simulink model "gm_current_fpga_slrt"  (R2020b)
settings: Solver=FixedStepAuto  StartTime=0.0  StopTime=10.0  RelTol=1e-3
undefined symbols (not defined in the file): current_fpga, FPGA, IO334
libraries: speedgoatlib_hdlCoder_IO3xx x5
settings Model: SimulationMode=external  Creator=Student  LastModifiedBy=Student
settings SolverCC: ConcurrentTasks=on  PositivePriorityOrder=on
settings OptimizationCC: BlockReduction=off  ConditionallyExecuteInputs=off  DefaultParameterBehavior=Inlined  OptimizeBlockIOStorage=off
settings DebuggingCC: AlgebraicLoopMsg=error  TasksWithSamePriorityMsg=none
settings HardwareCC: ProdBitPerLong=64  ProdLongLongMode=on  ProdHWDeviceType=Intel->x86-64 (Linux 64)  TargetBitPerPointer=64  TargetBitPerSizeT=64  TargetBitPerPtrDiffT=64  TargetLongLongMode=on  TargetIntDivRoundTo=Zero  TargetEndianess=LittleEndian  TargetWordSize=64  TargetHWDeviceType=Custom Processor->MATLAB Host Computer
settings RTWCC: Description=Simulink Real-Time  SystemTargetFile=slrealtime.tlc  TemplateMakefile=slrealtime_default_tmf  Toolchain=Simulink Real-Time Toolchain  BuildConfiguration=Faster Runs  CodeExecutionProfiling=on  TargetLang=C++

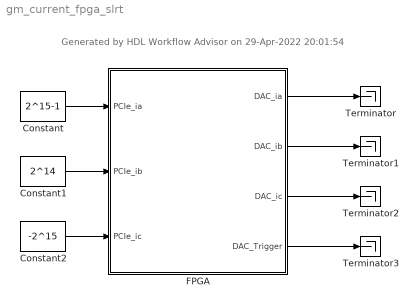
== system gm_current_fpga_slrt ==
  note: Generated by HDL Workflow Advisor on 29-Apr-2022 20:01:54
  Constant : Constant  Value=2^15-1  OutDataTypeStr=int16  SampleTime=5e-5
  Constant1 : Constant  Value=2^14  OutDataTypeStr=int16  SampleTime=5e-5
  Constant2 : Constant  Value=-2^15  OutDataTypeStr=int16  SampleTime=5e-5
  FPGA : Subsystem  mask(Speedgoat IO334-325k Interface Block){module_id=1, slot=-1, ts=-1, OutputRange=Auto (same as ADC), FpgaFreq=100}
      mask prompts: module_id "FPGA Module Identifier:"; slot "PCI slot (-1: autosearch):"; ts "Sample time:"; OutputRange "DAC Voltage Range:"; FpgaFreq "FPGA Frequency [MHz]"
      mask help: Simulink Real-Time Interface Block for Speedgoat IO334-325k.
      mask init:
      | hdlslrt.backend.mfpgaparameters;
      mask Help: eval('speedgoatdoc_hdlc')
      mask TypeOptions OutputRange: IO334 DAC Setup/OutputRange
      mask DialogControl AnalogOutput Prompt: Analog Output
      mask Display:
      | SetupBlkPath = find_system(gcb, 'LookUnderMasks', 'all', 'FollowLinks', 'on', 'regexp', 'on', 'Name', 'IO3(\d|x){2}\s+Setup' );
      | SetupBlkPath = SetupBlkPath{1};
      | TS = get_param(SetupBlkPath,'timestamp_mcs');
      | disp(sprintf('Speedgoat IO334-325k\nFPGA I/O Module\n\nTimestamp\n%s\n\nReference Design\nVersion 2.1\n\nMatlab R2020b\n\nPCIe Link Width: X4\nRear Plugin: -21\nAurora Mode: None\nAurora Byteswap: true\n', TS))
  Terminator{,1..3} (4 alike) : Terminator
  wires:
  Constant1/1 -> FPGA/2(PCIe_ib)
  Constant2/1 -> FPGA/3(PCIe_ic)
  Constant/1 -> FPGA/1(PCIe_ia)
  FPGA/2(DAC_ib) -> Terminator1/1
  FPGA/3(DAC_ic) -> Terminator2/1
  FPGA/4(DAC_Trigger) -> Terminator3/1
  FPGA/1(DAC_ia) -> Terminator/1

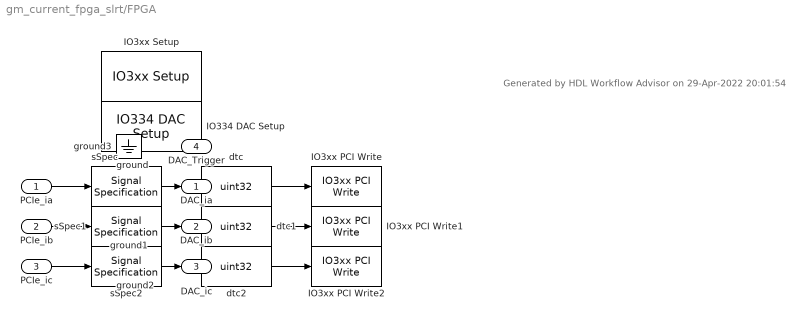
== system gm_current_fpga_slrt/FPGA ==
  note: Generated by HDL Workflow Advisor on 29-Apr-2022 20:01:54
  PCIe_ia : Inport
  PCIe_ib : Inport  Port=2
  PCIe_ic : Inport  Port=3
  IO334 DAC Setup : speedgoatlib_hdlCoder_IO3xx/IO334 DAC Setup  module_id=module_id  OutputRange=Auto (same as ADC)
  IO3xx PCI Write : speedgoatlib_hdlCoder_IO3xx/IO3xx PCI Write  device_id=1  module_id=module_id  board_type=IO334-325k  port_name=PCIe_ia  port_offset=hex2dec('100')  port_type=uint32  port_dim=1  strobe=0  sample_time=ts
  IO3xx PCI Write1 : speedgoatlib_hdlCoder_IO3xx/IO3xx PCI Write  device_id=1  module_id=module_id  board_type=IO334-325k  port_name=PCIe_ib  port_offset=hex2dec('104')  port_type=uint32  port_dim=1  strobe=0  sample_time=ts
  IO3xx PCI Write2 : speedgoatlib_hdlCoder_IO3xx/IO3xx PCI Write  device_id=1  module_id=module_id  board_type=IO334-325k  port_name=PCIe_ic  port_offset=hex2dec('108')  port_type=uint32  port_dim=1  strobe=0  sample_time=ts
  IO3xx Setup : speedgoatlib_hdlCoder_IO3xx/IO3xx Setup  mdl_ss_name=current_fpga/FPGA  board_type=IO334-325k  fpga_sync_mode=on  reset_mode=on  device_id=1  module_id=module_id  pci_slot=slot  fpga_mat_file=hdl_prj\hdlsrc\current_fpga\FPGA.mat  timestamp_mcs=04/29/22 19:36:43  timestamp=2204291832  tsreg=hex2dec('8')  bsf_file=FPGA_2204291832.mcs  mcs=0
  dtc : DataTypeConversion  OutDataTypeStr=uint32  ConvertRealWorld=Stored Integer (SI)  RndMeth=Zero
  dtc1 : DataTypeConversion  OutDataTypeStr=uint32  ConvertRealWorld=Stored Integer (SI)  RndMeth=Zero
  dtc2 : DataTypeConversion  OutDataTypeStr=uint32  ConvertRealWorld=Stored Integer (SI)  RndMeth=Zero
  ground{,1..3} (4 alike) : Ground
  sSpec : SignalSpecification  OutDataTypeStr=fixdt(1,16,0)
  sSpec1 : SignalSpecification  OutDataTypeStr=fixdt(1,16,0)
  sSpec2 : SignalSpecification  OutDataTypeStr=fixdt(1,16,0)
  DAC_ia : Outport
  DAC_ib : Outport  Port=2
  DAC_ic : Outport  Port=3
  DAC_Trigger : Outport  Port=4
  wires:
  PCIe_ia/1 -> sSpec/1
  sSpec/1 -> dtc/1
  dtc/1 -> IO3xx PCI Write/1
  PCIe_ib/1 -> sSpec1/1
  sSpec1/1 -> dtc1/1
  dtc1/1 -> IO3xx PCI Write1/1
  PCIe_ic/1 -> sSpec2/1
  sSpec2/1 -> dtc2/1
  dtc2/1 -> IO3xx PCI Write2/1
  ground/1 -> DAC_ia/1
  ground1/1 -> DAC_ib/1
  ground2/1 -> DAC_ic/1
  ground3/1 -> DAC_Trigger/1
